simulink library "LopesDevelopmentLibrary"  (R2015b)
settings: Solver=ode45  StartTime=0.0  StopTime=10.0  RelTol=1e-3
values from neighbouring files (symbols this model uses):
  d2r = @(d) d*(pi/180)    [LopesDevelopmentLibrary_LoadParameters.m]
  ts = LopesParams.ts    [LopesDevelopmentLibrary_LoadParameters.m]
undefined symbols (not defined in the file or in its folder): anyParameterChanged, DiscIntNeverNeededParam, gcbh, LAP, LHF, LKF, LopesParams, macaddr, mxpcnetworkconfig, mxpcrtudprx, mxpcrtudptx, patientParametersChanged, port, PX, PZ, RAP, RHF, RKF, SelectorLOPESInSize, StrideTime_s, Time
undefined symbols (not defined in the file): LopesParamsSendDataArrayLen
libraries: LopesDevelopmentLibrary x327, simulink x100, dspmtrx3 x49, xpciplib x6, xpcnetworkbufferlib x5, dspsigops x4, dspstat3 x3, xpcethernetlib x2, visionstatistics x2, xpcseriallib x2, LopesDevelopmentLibraryTest x1, nmc x1
(part 6 of 12)

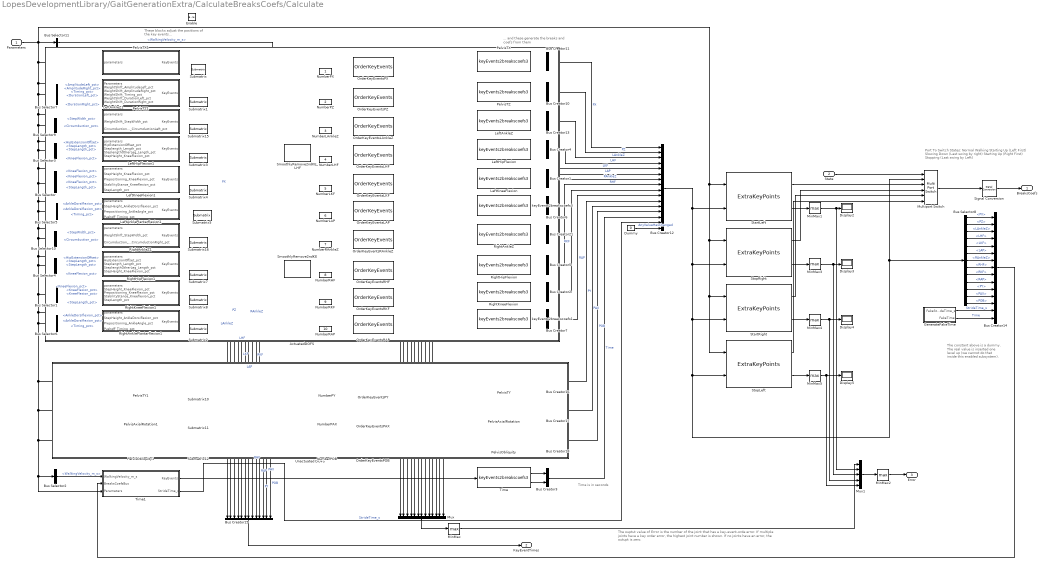
== system LopesDevelopmentLibrary/GaitGenerationExtra/CalculateBreaksCoefs/Calculate ==
  note: The ouptut value of Error is the number of the joint that has a key-event-orde  error.
      | If multiple joints have a key order error, the highest joint number is shown. If
      | no joints have an error, the outupt is zero.
  note: The constant above is
      | a dummy. The real value
      | is inserted one level up
      | (we cannot do that inside this
      | enabled subsystem).
  note: These blocks adjust the positions
      | of the key events...
  note: ... and these generate the breaks
      | and coefs from them
  note: Time is in seconds
  note: Port To Switch States:
      | Normal Walking
      | Starting Up (Left First)
      | Slowing Down (Last swing by right)
      | Starting Up (Right First)
      | Stopping (Last swing by Left)
  Parameters : Inport
  State : Inport  Port=2
  Enable : EnablePort
  ActuatedDOFS : Subsystem
      mask Display: disp('')
  Bus Creator{1..7,10..11,13,16..18,21} (14 alike) : BusCreator  Inputs=2
  Bus Creator12 : BusCreator  Inputs=16
  Bus Creator14 : BusCreator  Inputs=15
  Bus Creator15 : BusCreator  Inputs=13
  Bus Selector : BusSelector  OutputSignals=LeftStepHeight.KneeFlexion_pct,LeftPrepositioning.KneeFlexion_pct,LeftStabilityStance.KneeFlexion_pct,LeftSteplength.StepLength_pct
  Bus Selector1 : BusSelector  OutputSignals=RightStepHeight.KneeFlexion_pct,RightPrepositioning.KneeFlexion_pct,RightStabilityStance.KneeFlexion_pct,RightSteplength.StepLength_pct
  Bus Selector10 : BusSelector  OutputSignals=WeightShift.StepWidth_pct,RightCircumduction.Circumduction_pct
  Bus Selector11 : BusSelector  OutputSignals=General.WalkingVelocity_m_s
  Bus Selector2 : BusSelector  OutputSignals=General.WalkingVelocity_m_s
  Bus Selector3 : BusSelector  OutputSignals=General.HipExtensionOffset,LeftSteplength.StepLength_pct,RightSteplength.StepLength_pct,LeftStepHeight.KneeFlexion_pct
  Bus Selector4 : BusSelector  OutputSignals=General.HipExtensionOffset,RightSteplength.StepLength_pct,LeftSteplength.StepLength_pct,RightStepHeight.KneeFlexion_pct
  Bus Selector5 : BusSelector  OutputSignals=LeftStepHeight.AnkleDorsiflexion_pct,LeftPrepositioning.AnkleDorsiflexion_pct,LeftPushoff.Timing_pct
  Bus Selector6 : BusSelector  OutputSignals=RightStepHeight.AnkleDorsiflexion_pct,RightPrepositioning.AnkleDorsiflexion_pct,RightPushoff.Timing_pct
  Bus Selector7 : BusSelector  OutputSignals=WeightShift.AmplitudeLeft_pct,WeightShift.AmplitudeRight_pct,WeightShift.Timing_pct,WeightShift.DurationLeft_pct,WeightShift.DurationRight_pct
  Bus Selector8 : BusSelector  OutputSignals=PX,PZ,LAnkleZ,LHF,LKF,LAP,RAnkleZ,RHF,RKF,RAP,PY,PAX,POB
  Bus Selector9 : BusSelector  OutputSignals=WeightShift.StepWidth_pct,LeftCircumduction.Circumduction_pct
  Display{2..5} (4 alike) : Display
  Dummy : Constant  Value=0  OutDataTypeStr=double
  GenerateFakeTime : Subsystem
  LeftAnklePlantarflexion1 : Subsystem
  LeftAnkleZ : LopesDevelopmentLibrary/BlocksForInternalUse/GaitGeneration/keyEvents2breakscoefs3  SystemSampleTime=-1
  LeftAnkleZ1 : Subsystem
  LeftHipFlexion : LopesDevelopmentLibrary/BlocksForInternalUse/GaitGeneration/keyEvents2breakscoefs3  SystemSampleTime=-1
  LeftHipFlexion1 : Subsystem
  LeftKneeFlexion : LopesDevelopmentLibrary/BlocksForInternalUse/GaitGeneration/keyEvents2breakscoefs3  SystemSampleTime=-1
  LeftKneeFlexion1 : Subsystem
  MinMax{,1..5} (6 alike) : MinMax  Function=max
  Multiport Switch : MultiPortSwitch  Inputs=5
  Mux : Mux  Inputs=13
  Mux1 : Mux  Inputs=5
  NumberLAP : Constant  Value=6
  NumberLAnkleZ : Constant  Value=3
  NumberLHF : Constant  Value=4
  NumberLKF : Constant  Value=5
  NumberPAX : Constant  Value=12
  NumberPOB : Constant  Value=13
  NumberPX : Constant
  NumberPY : Constant  Value=11
  NumberPZ : Constant  Value=2
  NumberRAP : Constant  Value=10
  NumberRAnkleZ : Constant  Value=7
  NumberRHF : Constant  Value=8
  NumberRKF : Constant  Value=9
  OrderKeyEventsLAP : LopesDevelopmentLibrary/BlocksForInternalUse/GaitGeneration/OrderKeyEvents
  OrderKeyEventsLAnkleZ : LopesDevelopmentLibrary/BlocksForInternalUse/GaitGeneration/OrderKeyEvents
  OrderKeyEventsLHF : LopesDevelopmentLibrary/BlocksForInternalUse/GaitGeneration/OrderKeyEvents
  OrderKeyEventsLKF : LopesDevelopmentLibrary/BlocksForInternalUse/GaitGeneration/OrderKeyEvents
  OrderKeyEventsPAX : LopesDevelopmentLibrary/BlocksForInternalUse/GaitGeneration/OrderKeyEvents
  OrderKeyEventsPOB : LopesDevelopmentLibrary/BlocksForInternalUse/GaitGeneration/OrderKeyEvents
  OrderKeyEventsPX : LopesDevelopmentLibrary/BlocksForInternalUse/GaitGeneration/OrderKeyEvents
  OrderKeyEventsPY : LopesDevelopmentLibrary/BlocksForInternalUse/GaitGeneration/OrderKeyEvents
  OrderKeyEventsPZ : LopesDevelopmentLibrary/BlocksForInternalUse/GaitGeneration/OrderKeyEvents
  OrderKeyEventsRAP : LopesDevelopmentLibrary/BlocksForInternalUse/GaitGeneration/OrderKeyEvents
  OrderKeyEventsRAnkleZ : LopesDevelopmentLibrary/BlocksForInternalUse/GaitGeneration/OrderKeyEvents
  OrderKeyEventsRHF : LopesDevelopmentLibrary/BlocksForInternalUse/GaitGeneration/OrderKeyEvents
  OrderKeyEventsRKF : LopesDevelopmentLibrary/BlocksForInternalUse/GaitGeneration/OrderKeyEvents
  PelvisAxialRotation : LopesDevelopmentLibrary/BlocksForInternalUse/GaitGeneration/keyEvents2breakscoefs3  SystemSampleTime=-1
  PelvisAxialRotation1 : Subsystem
  PelvisObliquity : LopesDevelopmentLibrary/BlocksForInternalUse/GaitGeneration/keyEvents2breakscoefs3  SystemSampleTime=-1
  PelvisObliquity1 : Subsystem
  PelvisTX : LopesDevelopmentLibrary/BlocksForInternalUse/GaitGeneration/keyEvents2breakscoefs3  SystemSampleTime=-1
  PelvisTX1 : Subsystem
  PelvisTY : LopesDevelopmentLibrary/BlocksForInternalUse/GaitGeneration/keyEvents2breakscoefs3  SystemSampleTime=-1
  PelvisTY1 : Subsystem
  PelvisTZ : LopesDevelopmentLibrary/BlocksForInternalUse/GaitGeneration/keyEvents2breakscoefs3  SystemSampleTime=-1
  PelvisTZ1 : Subsystem
  RightAnklePlantarflexion1 : Subsystem
  RightAnkleZ : LopesDevelopmentLibrary/BlocksForInternalUse/GaitGeneration/keyEvents2breakscoefs3  SystemSampleTime=-1
  RightAnkleZ1 : Subsystem
  RightHipFlexion : LopesDevelopmentLibrary/BlocksForInternalUse/GaitGeneration/keyEvents2breakscoefs3  SystemSampleTime=-1
  RightHipFlexion1 : Subsystem
  RightKneeFlexion : LopesDevelopmentLibrary/BlocksForInternalUse/GaitGeneration/keyEvents2breakscoefs3  SystemSampleTime=-1
  RightKneeFlexion1 : Subsystem
  Signal Conversion : SignalConversion
  SmoothlyRemove2ndKE : LopesDevelopmentLibrary/BlocksForInternalUse/GaitGeneration/SmoothlyRemove2ndKE
  SmoothlyRemove2ndKE_LHF : LopesDevelopmentLibrary/BlocksForInternalUse/GaitGeneration/SmoothlyRemove2ndKE
  StartLeft : LopesDevelopmentLibrary/BlocksForInternalUse/GaitGenerationStartStop/ExtraKeyPoints   ExtraData='StartLeft'  ConnectionPoint=100  SetVelocity=0.3  SetStrideTime=2
  StartRight : LopesDevelopmentLibrary/BlocksForInternalUse/GaitGenerationStartStop/ExtraKeyPoints   ExtraData='StartRight'  ConnectionPoint=50  SetVelocity=0.3  SetStrideTime=2
  StopLeft : LopesDevelopmentLibrary/BlocksForInternalUse/GaitGenerationStartStop/ExtraKeyPoints   ExtraData='StopLeft'  ConnectionPoint=50  SetVelocity=0.3  SetStrideTime=2
  StopRight : LopesDevelopmentLibrary/BlocksForInternalUse/GaitGenerationStartStop/ExtraKeyPoints   ExtraData='StopRight'  ConnectionPoint=100  SetVelocity=0.3  SetStrideTime=2
  Submatrix{,1..5,7..8,10..12,15..16} (13 alike) : dspmtrx3/Submatrix  RowSpan=All rows  RowStartMode=First  RowStartIndex=1  RowEndMode=Last  RowEndIndex=1  ColSpan=One column  ColStartMode=First  ColStartIndex=1  ColEndMode=Last  ColEndIndex=1
  Time : LopesDevelopmentLibrary/BlocksForInternalUse/GaitGeneration/keyEvents2breakscoefs3  SystemSampleTime=-1
  Time1 : Subsystem
  Unactuated DOFS : Subsystem
      mask Display: disp('')
  keyEvents2breakscoefs1 : LopesDevelopmentLibrary/BlocksForInternalUse/GaitGeneration/keyEvents2breakscoefs3  SystemSampleTime=-1
  keyEvents2breakscoefs3 : LopesDevelopmentLibrary/BlocksForInternalUse/GaitGeneration/keyEvents2breakscoefs3  SystemSampleTime=-1
  BreaksCoefs : Outport  InitialOutput=0
  KeyEventTimes : Outport  Port=2
  Error : Outport  Port=3
  wires:
  Signal Conversion/1 -> BreaksCoefs/1
  OrderKeyEventsRKF/1 -> RightKneeFlexion/1
  OrderKeyEventsLHF/1 -> LeftHipFlexion/1
  Bus Selector7/5 -> PelvisTZ1/6(WeightShift_DurationRight_pct)  "<DurationRight_pct>"
  LeftHipFlexion1/1(KeyEvents) -> SmoothlyRemove2ndKE_LHF/1, Submatrix3/1
  LeftKneeFlexion/2 -> Bus Creator1/2
  LeftHipFlexion/1 -> Bus Creator4/1
  NumberRHF/1 -> OrderKeyEventsRHF/2
  LeftKneeFlexion/1 -> Bus Creator1/1
  MinMax/1 -> Mux1/1
  NumberRAnkleZ/1 -> OrderKeyEventsRAnkleZ/2
  OrderKeyEventsPOB/1 -> PelvisObliquity/1
  NumberLHF/1 -> OrderKeyEventsLHF/2
  OrderKeyEventsPY/1 -> PelvisTY/1
  NumberPZ/1 -> OrderKeyEventsPZ/2
  OrderKeyEventsPAX/1 -> PelvisAxialRotation/1
  LeftHipFlexion/2 -> Bus Creator4/2
  NumberLKF/1 -> OrderKeyEventsLKF/2
  Bus Selector3/4 -> LeftHipFlexion1/5(StepHeight_KneeFlexion_pct)  "<KneeFlexion_pct>"
  NumberRKF/1 -> OrderKeyEventsRKF/2
  Bus Selector3/3 -> LeftHipFlexion1/4(SteplengthOtherLeg_Length_pct)  "<StepLength_pct>"
  Bus Selector3/2 -> LeftHipFlexion1/3(Steplength_Length_pct)  "<StepLength_pct>"
  Dummy/1 -> Bus Creator12/16  "AnyValueHasChanged"
  RightHipFlexion1/1(KeyEvents) -> Submatrix7/1, SmoothlyRemove2ndKE/1
  RightKneeFlexion1/1(KeyEvents) -> OrderKeyEventsRKF/1, Submatrix8/1
  PelvisTX/2 -> Bus Creator11/2
  Bus Creator2/1 -> Bus Creator12/9  "RKF"
  PelvisTX/1 -> Bus Creator11/1
  Bus Creator1/1 -> Bus Creator12/5  "LKF"
  RightHipFlexion/2 -> Bus Creator5/2
  GenerateFakeTime/1(FakeStrideTime_s) -> Bus Creator14/14  "StrideTime_s"
  Bus Selector7/3 -> PelvisTZ1/4(WeightShift_Timing_pct)  "<Timing_pct>"
  LeftKneeFlexion1/1(KeyEvents) -> OrderKeyEventsLKF/1, Submatrix4/1
  Bus Selector7/1 -> PelvisTZ1/2(WeightShift_AmplitudeLeft_pct)  "<AmplitudeLeft_pct>"
  Bus Creator5/1 -> Bus Creator12/8  "RHF"
  Bus Selector7/4 -> PelvisTZ1/5(WeightShift_DurationLeft_pct)  "<DurationLeft_pct>"
  Bus Selector/1 -> LeftKneeFlexion1/2(StepHeight_KneeFlexion_pct)  "<KneeFlexion_pct>"
  Bus Selector4/4 -> RightHipFlexion1/5(StepHeight_KneeFlexion_pct)  "<KneeFlexion_pct>"
  PelvisTX1/1(KeyEvents) -> Submatrix/1, OrderKeyEventsPX/1
  Bus Creator15/1 -> KeyEventTimes/1
  Bus Creator10/1 -> Bus Creator12/2  "PZ"
  Bus Creator11/1 -> Bus Creator12/1  "PX"
  Bus Creator4/1 -> Bus Creator12/4  "LHF"
  Bus Selector4/3 -> RightHipFlexion1/4(SteplengthOtherLeg_Length_pct)  "<StepLength_pct>"
  Bus Selector4/2 -> RightHipFlexion1/3(Steplength_Length_pct)  "<StepLength_pct>"
  PelvisTZ1/1(KeyEvents) -> OrderKeyEventsPZ/1, Submatrix1/1
  PelvisTZ/1 -> Bus Creator10/1
  PelvisTZ/2 -> Bus Creator10/2
  Bus Selector1/4 -> RightKneeFlexion1/5(StepLength_pct)  "<StepLength_pct>"
  SmoothlyRemove2ndKE/1 -> OrderKeyEventsRHF/1
  Bus Selector4/1 -> RightHipFlexion1/2(HipExtensionOffset_pct)  "<HipExtensionOffset>"
  Submatrix10/1 -> Bus Creator15/11  "PY"
  Time1/2(StrideTime_s) -> Bus Creator12/15  "StrideTime_s"
  SmoothlyRemove2ndKE_LHF/1 -> OrderKeyEventsLHF/1
  Bus Selector3/1 -> LeftHipFlexion1/2(HipExtensionOffset_pct)  "<HipExtensionOffset>"
  Bus Selector1/3 -> RightKneeFlexion1/4(StabilityStance_Kneeflexion_pct)  "<KneeFlexion_pct>"
  Bus Selector1/1 -> RightKneeFlexion1/2(StepHeight_KneeFlexion_pct)  "<KneeFlexion_pct>"
  Bus Selector9/2 -> LeftAnkleZ1/3(Circumduction_CircumductionLeft_pct)  "<Circumduction_pct>"
  Bus Selector9/1 -> LeftAnkleZ1/2(WeightShift_StepWidth_pct)  "<StepWidth_pct>"
  NumberLAnkleZ/1 -> OrderKeyEventsLAnkleZ/2
  Bus Selector8/1 -> Bus Creator14/1  "<PX>"
  Bus Selector10/1 -> RightAnkleZ1/2(WeightShift_StepWidth_pct)  "<StepWidth_pct>"
  NumberPX/1 -> OrderKeyEventsPX/2
  Bus Selector10/2 -> RightAnkleZ1/3(Circumduction_CircumductionRight_pct)  "<Circumduction_pct>"
  Bus Selector/4 -> LeftKneeFlexion1/5(StepLength_pct)  "<StepLength_pct>"
  OrderKeyEventsRAnkleZ/1 -> RightAnkleZ/1
  Bus Creator21/1 -> Bus Creator12/7  "RAnkleZ"
  Bus Selector1/2 -> RightKneeFlexion1/3(Prepositioning_KneeFlexion_pct)  "<KneeFlexion_pct>"
  Mux/1 -> MinMax/1
  Bus Selector7/2 -> PelvisTZ1/3(WeightShift_AmplitudeRight_pct)  "<AmplitudeRight_pct>"
  Bus Selector/2 -> LeftKneeFlexion1/3(Prepositioning_KneeFlexion_pct)  "<KneeFlexion_pct>"
  Bus Creator13/1 -> Bus Creator12/3  "LAnkleZ"
  Bus Selector8/2 -> Bus Creator14/2  "<PZ>"
  Bus Selector/3 -> LeftKneeFlexion1/4(StabilityStance_Kneeflexion_pct)  "<KneeFlexion_pct>"
  Bus Selector8/8 -> Bus Creator14/8  "<RHF>"
  LeftAnkleZ/2 -> Bus Creator13/2
  LeftAnkleZ1/1(KeyEvents) -> Submatrix15/1, OrderKeyEventsLAnkleZ/1
  LeftAnkleZ/1 -> Bus Creator13/1
  RightAnkleZ/2 -> Bus Creator21/2
  RightAnkleZ/1 -> Bus Creator21/1
  RightAnkleZ1/1(KeyEvents) -> Submatrix16/1, OrderKeyEventsRAnkleZ/1
  Bus Selector8/12 -> Bus Creator14/12  "<PAX>"
  OrderKeyEventsLAnkleZ/1 -> LeftAnkleZ/1
  Submatrix11/1 -> Bus Creator15/12  "PAX"
  Time/1 -> Bus Creator3/1
  PelvisTY/1 -> Bus Creator16/1
  Bus Selector8/4 -> Bus Creator14/4  "<LHF>"
  Bus Selector8/7 -> Bus Creator14/7  "<RAnkleZ>"
  Bus Selector8/11 -> Bus Creator14/11  "<PY>"
  OrderKeyEventsLAnkleZ/2 -> Mux/3
  Bus Selector8/13 -> Bus Creator14/13  "<POB>"
  Submatrix12/1 -> Bus Creator15/13  "POB"
  Bus Selector8/9 -> Bus Creator14/9  "<RKF>"
  Submatrix8/1 -> Bus Creator15/9  "RKF"
  Submatrix7/1 -> Bus Creator15/8  "RHF"
  Bus Selector8/5 -> Bus Creator14/5  "<LKF>"
  PelvisObliquity1/1(KeyEvents) -> Submatrix12/1, OrderKeyEventsPOB/1
  Bus Selector11/1 -> SmoothlyRemove2ndKE/2, SmoothlyRemove2ndKE_LHF/2  "<WalkingVelocity_m_s>"
  PelvisTY1/1(KeyEvents) -> OrderKeyEventsPY/1, Submatrix10/1
  OrderKeyEventsPZ/2 -> Mux/2
  Submatrix16/1 -> Bus Creator15/7  "RAnkleZ"
  GenerateFakeTime/2(FakeTime) -> Bus Creator14/15  "Time"
  OrderKeyEventsRHF/2 -> Mux/8
  NumberPOB/1 -> OrderKeyEventsPOB/2
  OrderKeyEventsLKF/2 -> Mux/5
  NumberPY/1 -> OrderKeyEventsPY/2
  OrderKeyEventsRAnkleZ/2 -> Mux/7
  Bus Creator16/1 -> Bus Creator12/11  "PY"
  Submatrix/1 -> Bus Creator15/1  "PX"
  Submatrix15/1 -> Bus Creator15/3  "LAnkleZ"
  Submatrix3/1 -> Bus Creator15/4  "LHF"
  Submatrix1/1 -> Bus Creator15/2  "PZ"
  OrderKeyEventsLHF/2 -> Mux/4
  Submatrix4/1 -> Bus Creator15/5  "LKF"
  OrderKeyEventsRKF/2 -> Mux/9
  OrderKeyEventsPY/2 -> Mux/11
  OrderKeyEventsPOB/2 -> Mux/13
  OrderKeyEventsPX/2 -> Mux/1
  OrderKeyEventsPAX/2 -> Mux/12
  Bus Selector8/3 -> Bus Creator14/3  "<LAnkleZ>"
  PelvisTY/2 -> Bus Creator16/2
  OrderKeyEventsRHF/1 -> RightHipFlexion/1
  Time/2 -> Bus Creator3/2
  Bus Creator14/1 -> Time1/2(BreaksCoefsBus)
  RightHipFlexion/1 -> Bus Creator5/1
  OrderKeyEventsPX/1 -> PelvisTX/1
  OrderKeyEventsLKF/1 -> LeftKneeFlexion/1
  OrderKeyEventsPZ/1 -> PelvisTZ/1
  RightKneeFlexion/1 -> Bus Creator2/1
  Time1/1(KeyEvents) -> Time/1
  Bus Selector2/1 -> Time1/1(WalkingVelocity_m_s)  "<WalkingVelocity_m_s>"
  RightKneeFlexion/2 -> Bus Creator2/2
  PelvisObliquity/2 -> Bus Creator18/2
  Bus Creator17/1 -> Bus Creator12/12  "PAX"
  PelvisAxialRotation1/1(KeyEvents) -> Submatrix11/1, OrderKeyEventsPAX/1
  PelvisAxialRotation/2 -> Bus Creator17/2
  PelvisAxialRotation/1 -> Bus Creator17/1
  NumberPAX/1 -> OrderKeyEventsPAX/2
  Bus Creator18/1 -> Bus Creator12/13  "POB"
  PelvisObliquity/1 -> Bus Creator18/1
  Bus Creator3/1 -> Bus Creator12/14  "Time"
  OrderKeyEventsLAP/1 -> keyEvents2breakscoefs3/1
  OrderKeyEventsRAP/1 -> keyEvents2breakscoefs1/1
  keyEvents2breakscoefs3/1 -> Bus Creator6/1
  keyEvents2breakscoefs3/2 -> Bus Creator6/2
  Bus Creator6/1 -> Bus Creator12/6  "LAP"
  keyEvents2breakscoefs1/2 -> Bus Creator7/2
  keyEvents2breakscoefs1/1 -> Bus Creator7/1
  Bus Creator7/1 -> Bus Creator12/10  "RAP"
  Bus Selector8/10 -> Bus Creator14/10  "<RAP>"
  Bus Selector8/6 -> Bus Creator14/6  "<LAP>"
  OrderKeyEventsRAP/2 -> Mux/10
  OrderKeyEventsLAP/2 -> Mux/6
  NumberLAP/1 -> OrderKeyEventsLAP/2
  NumberRAP/1 -> OrderKeyEventsRAP/2
  RightAnklePlantarflexion1/1(KeyEvents) -> Submatrix2/1, OrderKeyEventsRAP/1
  Submatrix2/1 -> Bus Creator15/10  "RAP"
  LeftAnklePlantarflexion1/1(KeyEvents) -> OrderKeyEventsLAP/1, Submatrix5/1
  Submatrix5/1 -> Bus Creator15/6  "LAP"
  Bus Selector5/1 -> LeftAnklePlantarflexion1/2(StepHeight_AnkleDorsiflexion_pct)  "<AnkleDorsiflexion_pct>"
  Bus Selector5/2 -> LeftAnklePlantarflexion1/3(Prepositioning_AnkleAngle_pct)  "<AnkleDorsiflexion_pct>"
  Bus Selector5/3 -> LeftAnklePlantarflexion1/4(Pushoff_Timing_pct)  "<Timing_pct>"
  Bus Selector6/3 -> RightAnklePlantarflexion1/4(Pushoff_Timing_pct)  "<Timing_pct>"
  Bus Selector6/2 -> RightAnklePlantarflexion1/3(Prepositioning_AnkleAngle_pct)  "<AnkleDorsiflexion_pct>"
  Bus Selector6/1 -> RightAnklePlantarflexion1/2(StepHeight_AnkleDorsiflexion_pct)  "<AnkleDorsiflexion_pct>"
  MinMax5/1 -> Mux1/5, Display5/1
  MinMax4/1 -> Mux1/4, Display4/1
  StopLeft/2 -> MinMax5/1
  StartRight/2 -> MinMax4/1
  StopLeft/1 -> Multiport Switch/6
  StartRight/1 -> Multiport Switch/5
  StopRight/1 -> Multiport Switch/4
  MinMax3/1 -> Mux1/3, Display3/1
  StopRight/2 -> MinMax3/1
  StartLeft/1 -> Multiport Switch/3
  State/1 -> Multiport Switch/1
  MinMax1/1 -> Mux1/2, Display2/1
  StartLeft/2 -> MinMax1/1
  Parameters/1 -> Bus Selector11/1, StartLeft/1, StopRight/1, StartRight/1, StopLeft/1, Bus Selector5/1, RightAnklePlantarflexion1/1(parameters), Bus Selector6/1, Time1/3(Parameters), Bus Selector2/1, PelvisObliquity1/1(parameters), PelvisAxialRotation1/1(parameters), PelvisTY1/1(parameters), Bus Selector1/1, Bus Selector4/1, RightHipFlexion1/1(parameters), RightKneeFlexion1/1(parameters), Bus Selector10/1, RightAnkleZ1/1(parameters), LeftAnklePlantarflexion1/1(parameters), Bus Selector/1, LeftKneeFlexion1/1(parameters), Bus Selector3/1, LeftHipFlexion1/1(parameters), Bus Selector9/1, LeftAnkleZ1/1(parameters), Bus Selector7/1, PelvisTZ1/1(Parameters), PelvisTX1/1(parameters)
  Multiport Switch/1 -> Signal Conversion/1
  Mux1/1 -> MinMax2/1
  MinMax2/1 -> Error/1
  Bus Creator12/1 -> StartLeft/2, Bus Selector8/1, Multiport Switch/2, StopLeft/2, StartRight/2, StopRight/2

== system LopesDevelopmentLibrary/GaitGenerationExtra/GaitGenerationAndAnalysis/DesiredStateToSetState ==
  DesiredState : Inport
  Add : Sum  Inputs=5
  Add2 : Sum
  Compare To Constant1 : simulink/Logic and Bit Operations/Compare To Constant  relop=<  const=200  OutDataTypeStr=boolean
  Compare To Constant10 : simulink/Logic and Bit Operations/Compare To Constant  relop===  const=302  OutDataTypeStr=boolean
  Compare To Constant2 : simulink/Logic and Bit Operations/Compare To Constant  relop===  const=501  OutDataTypeStr=boolean
  Compare To Constant3 : simulink/Logic and Bit Operations/Compare To Constant  relop===  const=201  OutDataTypeStr=boolean
  Compare To Constant4 : simulink/Logic and Bit Operations/Compare To Constant  relop===  const=502  OutDataTypeStr=boolean
  Compare To Constant5 : simulink/Logic and Bit Operations/Compare To Constant  relop=>=  const=100  OutDataTypeStr=boolean
  Compare To Constant6 : simulink/Logic and Bit Operations/Compare To Constant  relop===  const=202  OutDataTypeStr=boolean
  Compare To Constant7 : simulink/Logic and Bit Operations/Compare To Constant  relop===  const=402  OutDataTypeStr=boolean
  Compare To Constant8 : simulink/Logic and Bit Operations/Compare To Constant  relop===  const=401  OutDataTypeStr=boolean
  Compare To Constant9 : simulink/Logic and Bit Operations/Compare To Constant  relop===  const=301  OutDataTypeStr=boolean
  Gain : Gain
  Gain1 : Gain  Gain=2
  Gain2 : Gain  Gain=4
  Gain3 : Gain  Gain=3
  Gain4 : Gain  Gain=5
  Gain7 : Gain  Gain=50  OutDataTypeStr=double
  Gain8 : Gain  Gain=0  OutDataTypeStr=double
  Logical Operator : Logic  AllPortsSameDT=off  OutDataTypeStr=boolean
  Logical Operator{1..10} (10 alike) : Logic  Operator=OR  AllPortsSameDT=off  OutDataTypeStr=boolean
  Unit Delay : UnitDelay  SampleTime=-1
  Unit Delay1 : UnitDelay  SampleTime=-1
  Unit Delay2 : UnitDelay  SampleTime=-1
  Unit Delay3 : UnitDelay  InitialCondition=2  SampleTime=-1
  Unit Delay4 : UnitDelay  InitialCondition=2  SampleTime=-1
  SetState : Outport
  Reset : Outport  Port=2
  ResetPercentage : Outport  Port=3
  FinalState : Outport  Port=4
  wires:
  Compare To Constant1/1 -> Logical Operator/2
  Compare To Constant5/1 -> Logical Operator/1
  Compare To Constant2/1 -> Logical Operator8/1, Logical Operator1/2
  Compare To Constant3/1 -> Logical Operator1/1
  Compare To Constant4/1 -> Logical Operator9/1, Logical Operator2/2
  Compare To Constant6/1 -> Logical Operator2/1
  Compare To Constant8/1 -> Logical Operator8/2, Logical Operator3/1
  Compare To Constant9/1 -> Logical Operator7/1, Logical Operator5/1, Logical Operator3/2
  Compare To Constant7/1 -> Logical Operator9/2, Logical Operator4/1
  DesiredState/1 -> Compare To Constant2/1, Compare To Constant1/1, Compare To Constant5/1, Compare To Constant3/1, Compare To Constant6/1, Compare To Constant7/1, Compare To Constant10/1, Compare To Constant9/1, Compare To Constant8/1, Compare To Constant4/1
  Compare To Constant10/1 -> Logical Operator7/2, Logical Operator6/2, Logical Operator4/2
  Logical Operator1/1 -> Gain1/1
  Logical Operator/1 -> Gain/1
  Logical Operator2/1 -> Gain2/1
  Logical Operator3/1 -> Gain3/1
  Logical Operator4/1 -> Gain4/1
  Gain/1 -> Add/1
  Gain1/1 -> Add/2
  Gain2/1 -> Add/3
  Gain3/1 -> Add/4
  Gain4/1 -> Add/5
  Add/1 -> Unit Delay4/1
  Logical Operator9/1 -> Logical Operator6/1, Logical Operator10/2
  Logical Operator8/1 -> Logical Operator10/1, Logical Operator5/2
  Unit Delay4/1 -> Unit Delay3/1
  Unit Delay3/1 -> SetState/1
  Gain8/1 -> Add2/2
  Gain7/1 -> Add2/1
  Logical Operator10/1 -> Unit Delay2/1
  Add2/1 -> Unit Delay/1
  Logical Operator5/1 -> Gain7/1
  Logical Operator6/1 -> Gain8/1
  Unit Delay/1 -> Unit Delay1/1
  Unit Delay1/1 -> ResetPercentage/1
  Unit Delay2/1 -> Reset/1
  Logical Operator7/1 -> FinalState/1

== system LopesDevelopmentLibrary/GaitGenerationExtra/GaitParameters/AssignChangedElements ==
  note: This block checks whether any of the parameters changed during
      | this sampletime, and assigns the correct values to the anyParameterChanged
      | and patientParametersChanged bus elements.
  BusIn : Inport
  PatientParametersChanged : Inport  Port=2
  AnyChanged : LopesDevelopmentLibrary/Various/AnyChanged
  Bus Assignment : BusAssignment  AssignedSignals=patientParametersChanged,anyParameterChanged
  Bus Selector : BusSelector  OutputSignals=Patient,General,WeightShift,LeftStepHeight,RightStepHeight,LeftCircumduction,RightCircumduction,LeftStabilityStance,RightStabilityStance,LeftPrepositioning,RightPrepositioning,LeftSteplength,RightSteplength  OutputAsBus=on
  Data Type Conversion2 : DataTypeConversion
  Logical Operator : Logic  Operator=OR  AllPortsSameDT=off  OutDataTypeStr=boolean
  BusOut : Outport
  Changed : Outport  Port=2
  wires:
  Data Type Conversion2/1 -> Changed/1
  Bus Assignment/1 -> BusOut/1
  Bus Selector/1 -> AnyChanged/1
  PatientParametersChanged/1 -> Logical Operator/1, Bus Assignment/2
  BusIn/1 -> Bus Selector/1, Bus Assignment/1
  Logical Operator/1 -> Bus Assignment/3, Data Type Conversion2/1
  AnyChanged/1 -> Logical Operator/2

== system LopesDevelopmentLibrary/GaitGenerationExtra/GaitParameters/Circumduction ==

== system LopesDevelopmentLibrary/GaitGenerationExtra/GaitParameters/General ==

== system LopesDevelopmentLibrary/GaitGenerationExtra/GaitParameters/Prepositioning ==

== system LopesDevelopmentLibrary/GaitGenerationExtra/GaitParameters/Pushoff ==

== system LopesDevelopmentLibrary/GaitGenerationExtra/GaitParameters/RateLimitCircumduction ==
  GeneralGF : Inport
  In2 : Inport  Port=2
  In3 : Inport  Port=3
  In4 : Inport  Port=4
  In5 : Inport  Port=5
  In6 : Inport  Port=6
  In7 : Inport  Port=7
  Bus Creator1 : BusCreator  Inputs=2
  Bus Creator2 : BusCreator  Inputs=2
  Rate Limiter : RateLimiter  RisingSlewLimit=100  FallingSlewLimit=-100  SampleTimeMode=inherited
  Rate Limiter1 : RateLimiter  RisingSlewLimit=50  FallingSlewLimit=-50  SampleTimeMode=inherited
  Rate Limiter2 : RateLimiter  RisingSlewLimit=50  FallingSlewLimit=-50  SampleTimeMode=inherited
  Rate Limiter7 : RateLimiter  RisingSlewLimit=100  FallingSlewLimit=-100  SampleTimeMode=inherited
  Switch : Switch  Criteria=u2 ~= 0
  Switch1 : Switch  Criteria=u2 ~= 0
  Left : Outport
  Right : Outport  Port=2
  wires:
  Bus Creator1/1 -> Left/1
  Rate Limiter1/1 -> Bus Creator1/2  "Circumduction_pct"
  Rate Limiter/1 -> Bus Creator1/1  "GuidanceForce_pct"
  Switch1/1 -> Rate Limiter7/1
  In2/1 -> Switch/2
  In6/1 -> Switch1/1
  In3/1 -> Switch/1
  In5/1 -> Switch1/2
  In7/1 -> Rate Limiter2/1
  Switch/1 -> Rate Limiter/1  "GuidanceForce_pct"
  In4/1 -> Rate Limiter1/1
  GeneralGF/1 -> Switch/3, Switch1/3
  Rate Limiter2/1 -> Bus Creator2/2  "Circumduction_pct"
  Rate Limiter7/1 -> Bus Creator2/1  "GuidanceForce_pct"
  Bus Creator2/1 -> Right/1

== system LopesDevelopmentLibrary/GaitGenerationExtra/GaitParameters/RateLimitGeneral ==
  In1 : Inport
  In2 : Inport  Port=2
  In3 : Inport  Port=3
  Bus Creator1 : BusCreator  Inputs=3
  ConvertToKm_h : Gain  Gain=3.6
  Rate Limiter1 : RateLimiter  RisingSlewLimit=50  FallingSlewLimit=-50  SampleTimeMode=inherited
  Rate Limiter2 : RateLimiter  RisingSlewLimit=0.1  FallingSlewLimit=-0.1  SampleTimeMode=inherited
  Rate Limiter3 : RateLimiter  RisingSlewLimit=20  FallingSlewLimit=-20  SampleTimeMode=inherited
  km_h : Outport
  General : Outport  Port=2
  wires:
  Bus Creator1/1 -> General/1  "General"
  In3/1 -> Rate Limiter1/1
  In2/1 -> Rate Limiter3/1
  In1/1 -> ConvertToKm_h/1, Rate Limiter2/1
  ConvertToKm_h/1 -> km_h/1
  Rate Limiter2/1 -> Bus Creator1/1  "WalkingVelocity_m_s"
  Rate Limiter3/1 -> Bus Creator1/2  "GuidanceForce_pct"
  Rate Limiter1/1 -> Bus Creator1/3  "HipExtensionOffset"

== system LopesDevelopmentLibrary/GaitGenerationExtra/GaitParameters/RateLimitPrepositioning ==
  GeneralGF : Inport
  In2 : Inport  Port=2
  In3 : Inport  Port=3
  In4 : Inport  Port=4
  In1 : Inport  Port=5
  In5 : Inport  Port=6
  In6 : Inport  Port=7
  In7 : Inport  Port=8
  In8 : Inport  Port=9
  Bus Creator1 : BusCreator  Inputs=3
  Bus Creator2 : BusCreator  Inputs=3
  Rate Limiter : RateLimiter  RisingSlewLimit=100  FallingSlewLimit=-100  SampleTimeMode=inherited
  Rate Limiter{1..4} (4 alike) : RateLimiter  RisingSlewLimit=50  FallingSlewLimit=-50  SampleTimeMode=inherited
  Rate Limiter7 : RateLimiter  RisingSlewLimit=100  FallingSlewLimit=-100  SampleTimeMode=inherited
  Switch : Switch  Criteria=u2 ~= 0
  Switch1 : Switch  Criteria=u2 ~= 0
  Left : Outport
  Right : Outport  Port=2
  wires:
  Bus Creator1/1 -> Left/1
  Rate Limiter1/1 -> Bus Creator1/2  "KneeFlexion_pct"
  Rate Limiter/1 -> Bus Creator1/1  "GuidanceForce_pct"
  Switch1/1 -> Rate Limiter7/1
  In2/1 -> Switch/2
  In6/1 -> Switch1/1
  In3/1 -> Switch/1
  In5/1 -> Switch1/2
  In7/1 -> Rate Limiter2/1
  Switch/1 -> Rate Limiter/1  "GuidanceForce_pct"
  In4/1 -> Rate Limiter1/1
  GeneralGF/1 -> Switch/3, Switch1/3
  Rate Limiter2/1 -> Bus Creator2/2  "KneeFlexion_pct"
  Rate Limiter7/1 -> Bus Creator2/1  "GuidanceForce_pct"
  Bus Creator2/1 -> Right/1
  Rate Limiter3/1 -> Bus Creator1/3  "AnkleDorsiflexion_pct"
  In1/1 -> Rate Limiter3/1
  Rate Limiter4/1 -> Bus Creator2/3  "AnkleDorsiflexion_pct"
  In8/1 -> Rate Limiter4/1

== system LopesDevelopmentLibrary/GaitGenerationExtra/GaitParameters/RateLimitPushoff ==
  GeneralGF : Inport
  In2 : Inport  Port=2
  In3 : Inport  Port=3
  In4 : Inport  Port=4
  In1 : Inport  Port=5
  In5 : Inport  Port=6
  In6 : Inport  Port=7
  In7 : Inport  Port=8
  In8 : Inport  Port=9
  Bus Creator1 : BusCreator  Inputs=3
  Bus Creator2 : BusCreator  Inputs=3
  Rate Limiter : RateLimiter  RisingSlewLimit=100  FallingSlewLimit=-100  SampleTimeMode=inherited
  Rate Limiter1 : RateLimiter  RisingSlewLimit=50  FallingSlewLimit=-50  SampleTimeMode=inherited
  Rate Limiter2 : RateLimiter  RisingSlewLimit=50  FallingSlewLimit=-50  SampleTimeMode=inherited
  Rate Limiter3 : RateLimiter  RisingSlewLimit=10  FallingSlewLimit=-10  SampleTimeMode=inherited
  Rate Limiter4 : RateLimiter  RisingSlewLimit=10  FallingSlewLimit=-10  SampleTimeMode=inherited
  Rate Limiter7 : RateLimiter  RisingSlewLimit=100  FallingSlewLimit=-100  SampleTimeMode=inherited
  Switch : Switch  Criteria=u2 ~= 0
  Switch1 : Switch  Criteria=u2 ~= 0
  Left : Outport
  Right : Outport  Port=2
  wires:
  In8/1 -> Rate Limiter4/1
  Rate Limiter4/1 -> Bus Creator2/3  "Timing_pct"
  In1/1 -> Rate Limiter3/1
  Rate Limiter3/1 -> Bus Creator1/3  "Timing_pct"
  Bus Creator2/1 -> Right/1
  Rate Limiter7/1 -> Bus Creator2/1  "GuidanceForce_pct"
  Rate Limiter2/1 -> Bus Creator2/2  "HipExtension_pct"
  GeneralGF/1 -> Switch1/3, Switch/3
  In4/1 -> Rate Limiter1/1
  Switch/1 -> Rate Limiter/1  "GuidanceForce_pct"
  In7/1 -> Rate Limiter2/1
  In5/1 -> Switch1/2
  In3/1 -> Switch/1
  In6/1 -> Switch1/1
  In2/1 -> Switch/2
  Switch1/1 -> Rate Limiter7/1
  Rate Limiter/1 -> Bus Creator1/1  "GuidanceForce_pct"
  Rate Limiter1/1 -> Bus Creator1/2  "HipExtension_pct"
  Bus Creator1/1 -> Left/1

== system LopesDevelopmentLibrary/GaitGenerationExtra/GaitParameters/RateLimitStabilityStance ==
  GeneralGF : Inport
  In2 : Inport  Port=2
  In3 : Inport  Port=3
  In4 : Inport  Port=4
  In5 : Inport  Port=5
  In6 : Inport  Port=6
  In7 : Inport  Port=7
  Bus Creator1 : BusCreator  Inputs=2
  Bus Creator2 : BusCreator  Inputs=2
  Rate Limiter : RateLimiter  RisingSlewLimit=100  FallingSlewLimit=-100  SampleTimeMode=inherited
  Rate Limiter1 : RateLimiter  RisingSlewLimit=50  FallingSlewLimit=-50  SampleTimeMode=inherited
  Rate Limiter2 : RateLimiter  RisingSlewLimit=50  FallingSlewLimit=-50  SampleTimeMode=inherited
  Rate Limiter7 : RateLimiter  RisingSlewLimit=100  FallingSlewLimit=-100  SampleTimeMode=inherited
  Switch : Switch  Criteria=u2 ~= 0
  Switch1 : Switch  Criteria=u2 ~= 0
  Left : Outport
  Right : Outport  Port=2
  wires:
  Bus Creator2/1 -> Right/1
  Rate Limiter7/1 -> Bus Creator2/1  "GuidanceForce_pct"
  Rate Limiter2/1 -> Bus Creator2/2  "KneeFlexion_pct"
  GeneralGF/1 -> Switch1/3, Switch/3
  In4/1 -> Rate Limiter1/1
  Switch/1 -> Rate Limiter/1  "GuidanceForce_pct"
  In7/1 -> Rate Limiter2/1
  In5/1 -> Switch1/2
  In3/1 -> Switch/1
  In6/1 -> Switch1/1
  In2/1 -> Switch/2
  Switch1/1 -> Rate Limiter7/1
  Rate Limiter/1 -> Bus Creator1/1  "GuidanceForce_pct"
  Rate Limiter1/1 -> Bus Creator1/2  "KneeFlexion_pct"
  Bus Creator1/1 -> Left/1

== system LopesDevelopmentLibrary/GaitGenerationExtra/GaitParameters/RateLimitStepHeight ==
  GeneralGF : Inport
  In2 : Inport  Port=2
  In3 : Inport  Port=3
  In1 : Inport  Port=4
  In4 : Inport  Port=5
  In5 : Inport  Port=6
  In6 : Inport  Port=7
  In8 : Inport  Port=8
  In7 : Inport  Port=9
  Bus Creator1 : BusCreator  Inputs=3
  Bus Creator2 : BusCreator  Inputs=3
  Rate Limiter : RateLimiter  RisingSlewLimit=100  FallingSlewLimit=-100  SampleTimeMode=inherited
  Rate Limiter1 : RateLimiter  RisingSlewLimit=50  FallingSlewLimit=-50  SampleTimeMode=inherited
  Rate Limiter2 : RateLimiter  RisingSlewLimit=50  FallingSlewLimit=-50  SampleTimeMode=inherited
  Rate Limiter3 : RateLimiter  RisingSlewLimit=100  FallingSlewLimit=-100  SampleTimeMode=inherited
  Rate Limiter4 : RateLimiter  RisingSlewLimit=50  FallingSlewLimit=-50  SampleTimeMode=inherited
  Rate Limiter7 : RateLimiter  RisingSlewLimit=100  FallingSlewLimit=-100  SampleTimeMode=inherited
  Switch : Switch  Criteria=u2 ~= 0
  Switch1 : Switch  Criteria=u2 ~= 0
  Left : Outport
  Right : Outport  Port=2
  wires:
  Bus Creator2/1 -> Right/1
  Rate Limiter7/1 -> Bus Creator2/1  "GuidanceForce_pct"
  Rate Limiter2/1 -> Bus Creator2/3  "KneeFlexion_pct"
  GeneralGF/1 -> Switch/3, Switch1/3
  In4/1 -> Rate Limiter1/1
  Switch/1 -> Rate Limiter/1  "GuidanceForce_pct"
  In7/1 -> Rate Limiter2/1
  In5/1 -> Switch1/2
  In3/1 -> Switch/1
  In6/1 -> Switch1/1
  In2/1 -> Switch/2
  Switch1/1 -> Rate Limiter7/1
  Rate Limiter/1 -> Bus Creator1/1  "GuidanceForce_pct"
  Rate Limiter1/1 -> Bus Creator1/3  "KneeFlexion_pct"
  Bus Creator1/1 -> Left/1
  Rate Limiter3/1 -> Bus Creator1/2  "AnkleDorsiflexion_pct"
  In1/1 -> Rate Limiter3/1
  Rate Limiter4/1 -> Bus Creator2/2  "AnkleDorsiflexion_pct"
  In8/1 -> Rate Limiter4/1

== system LopesDevelopmentLibrary/GaitGenerationExtra/GaitParameters/RateLimitStepLength ==
  GeneralGF : Inport
  In2 : Inport  Port=2
  In3 : Inport  Port=3
  In4 : Inport  Port=4
  Bus Creator1 : BusCreator  Inputs=2
  Rate Limiter : RateLimiter  RisingSlewLimit=100  FallingSlewLimit=-100  SampleTimeMode=inherited
  Rate Limiter1 : RateLimiter  RisingSlewLimit=5  FallingSlewLimit=-5  SampleTimeMode=inherited
  Switch : Switch  Criteria=u2 ~= 0
  StepLength : Outport
  wires:
  GeneralGF/1 -> Switch/3
  In4/1 -> Rate Limiter1/1
  Switch/1 -> Rate Limiter/1  "GuidanceForce_pct"
  In3/1 -> Switch/1
  In2/1 -> Switch/2
  Rate Limiter/1 -> Bus Creator1/1  "GuidanceForce_pct"
  Rate Limiter1/1 -> Bus Creator1/2  "StepLength_pct"
  Bus Creator1/1 -> StepLength/1

== system LopesDevelopmentLibrary/GaitGenerationExtra/GaitParameters/RateLimitWeightShift ==
  GeneralGF : Inport
  In2 : Inport  Port=2
  In3 : Inport  Port=3
  In4 : Inport  Port=4
  In5 : Inport  Port=5
  In6 : Inport  Port=6
  In7 : Inport  Port=7
  In8 : Inport  Port=8
  In9 : Inport  Port=9
  Bus Creator1 : BusCreator  Inputs=7
  Rate Limiter : RateLimiter  RisingSlewLimit=50  FallingSlewLimit=-50  SampleTimeMode=inherited
  Rate Limiter1 : RateLimiter  RisingSlewLimit=50  FallingSlewLimit=-50  SampleTimeMode=inherited
  Rate Limiter2 : RateLimiter  RisingSlewLimit=50  FallingSlewLimit=-50  SampleTimeMode=inherited
  Rate Limiter3 : RateLimiter  RisingSlewLimit=15  FallingSlewLimit=-15  SampleTimeMode=inherited
  Rate Limiter4 : RateLimiter  RisingSlewLimit=15  FallingSlewLimit=-15  SampleTimeMode=inherited
  Rate Limiter5 : RateLimiter  RisingSlewLimit=15  FallingSlewLimit=-15  SampleTimeMode=inherited
  Rate Limiter6 : RateLimiter  RisingSlewLimit=20  FallingSlewLimit=-20  SampleTimeMode=inherited
  Switch : Switch  Criteria=u2 ~= 0
  Out1 : Outport
  wires:
  In3/1 -> Switch/1
  Switch/1 -> Rate Limiter/1  "GuidanceForce_pct"
  In7/1 -> Rate Limiter4/1
  In8/1 -> Rate Limiter5/1
  In9/1 -> Rate Limiter6/1
  In4/1 -> Rate Limiter1/1
  In5/1 -> Rate Limiter2/1
  In6/1 -> Rate Limiter3/1
  GeneralGF/1 -> Switch/3
  Rate Limiter5/1 -> Bus Creator1/6  "DurationRight_pct"
  Rate Limiter/1 -> Bus Creator1/1  "GuidanceForce_pct"
  Rate Limiter4/1 -> Bus Creator1/5  "DurationLeft_pct"
  Rate Limiter3/1 -> Bus Creator1/4  "Timing_pct"
  Rate Limiter1/1 -> Bus Creator1/2  "AmplitudeLeft_pct"
  Rate Limiter6/1 -> Bus Creator1/7  "StepWidth_pct"
  Bus Creator1/1 -> Out1/1
  Rate Limiter2/1 -> Bus Creator1/3  "AmplitudeRight_pct"
  In2/1 -> Switch/2

== system LopesDevelopmentLibrary/GaitGenerationExtra/GaitParameters/StabilityInStance ==

== system LopesDevelopmentLibrary/GaitGenerationExtra/GaitParameters/StepHeight ==

== system LopesDevelopmentLibrary/GaitGenerationExtra/GaitParameters/StepLength ==

== system LopesDevelopmentLibrary/GaitGenerationExtra/GaitParameters/WeightShift ==

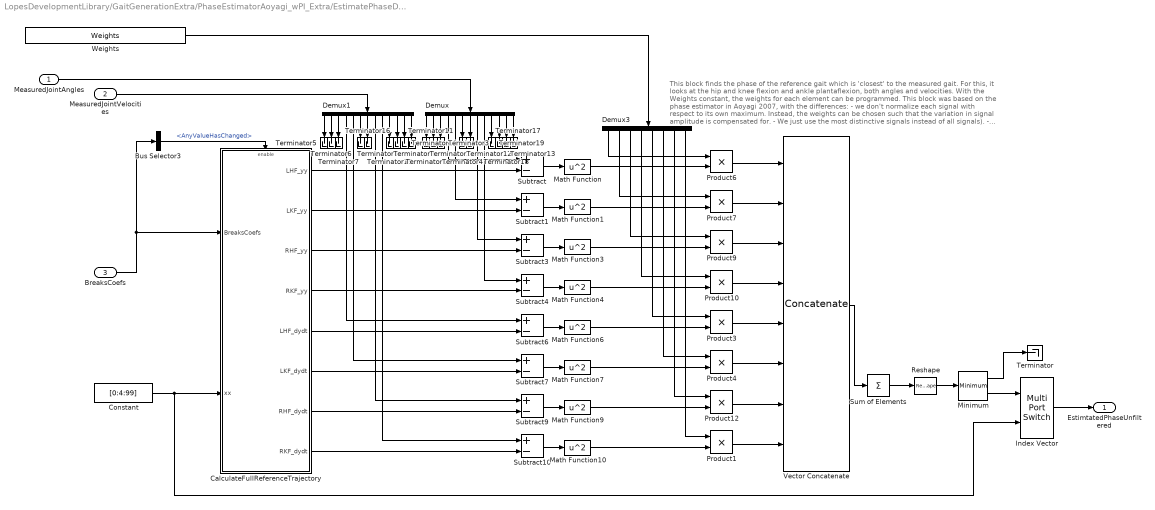
== system LopesDevelopmentLibrary/GaitGenerationExtra/PhaseEstimatorAoyagi_wPI_Extra/EstimatePhaseDirectlyAoyagi ==
  note: This block finds the phase of the reference gait which is 'closest' to the
      | measured gait. For this, it looks at the hip and knee flexion and ankle plantaflexion,
      | both angles and velocities. With the Weights constant, the weights for each element
      | can be programmed.
      | This block was based on the phase estimator in Aoyagi 2007, with the differences:
      | - we don't normalize each signal with respect to its own maximum. Instead, the weights
      | can be chosen such that the variation in signal amplitude is compensated for.
      | - We just use the most distinctive signals instead of all signals).
      | - The phase is expressed in percent  [0,100) instead of [0,1).
  MeasuredJointAngles : Inport
  MeasuredJointVelocities : Inport  Port=2
  BreaksCoefs : Inport  Port=3
  Bus Selector3 : BusSelector  OutputSignals=AnyValueHasChanged
  CalculateFullReferenceTrajectory : Subsystem
  Constant : Constant  Value=[0:4:99]
  Demux : Demux  Outputs=13
  Demux1 : Demux  Outputs=13
  Demux3 : Demux  Outputs=8
  Index Vector : MultiPortSwitch  Inputs=1
  Math Function{,1,3..4,6..7,9..10} (8 alike) : Math  Operator=square  SaturateOnIntegerOverflow=on
  Minimum : dspstat3/Minimum  fcn=Value and Index  reset=None  InputProcessing=Columns as channels (frame based)  indexBase=One  operateOver=Each column  Dimension=1  operation=minimum  roiEnable=off  roiType=Rectangles  roiPortion=Entire ROI  roiOutput=Individual statistics for each ROI  roiFlag=off  roundingMode=Floor  overflowMode=off
  Product{1,3..4,6..7,9..10,12} (8 alike) : Product  RndMeth=Zero
  Reshape : Reshape
  Subtract{,1,3..4,6..7,9..10} (8 alike) : Sum  Inputs=+-
  Sum of Elements : Sum  Inputs=+  CollapseMode=Specified dimension  CollapseDim=2
  Terminator{,1..13,15..19} (19 alike) : Terminator
  Vector Concatenate : Concatenate  NumInputs=8  Mode=Multidimensional array  ConcatenateDimension=2
  Weights : Constant  Value=Weights
  EstimtatedPhaseUnfiltered : Outport
  wires:
  Demux3/8 -> Product1/1
  Demux3/7 -> Product12/1
  Demux3/6 -> Product4/1
  Demux3/5 -> Product3/1
  Demux3/4 -> Product10/1
  Demux3/3 -> Product9/1
  Demux3/2 -> Product7/1
  Demux3/1 -> Product6/1
  Bus Selector3/1 -> CalculateFullReferenceTrajectory/Enable  "<AnyValueHasChanged>"
  CalculateFullReferenceTrajectory/8(RKF_dydt) -> Subtract10/2
  CalculateFullReferenceTrajectory/7(RHF_dydt) -> Subtract9/2
  CalculateFullReferenceTrajectory/6(LKF_dydt) -> Subtract7/2
  CalculateFullReferenceTrajectory/5(LHF_dydt) -> Subtract6/2
  CalculateFullReferenceTrajectory/4(RKF_yy) -> Subtract4/2
  CalculateFullReferenceTrajectory/3(RHF_yy) -> Subtract3/2
  CalculateFullReferenceTrajectory/2(LKF_yy) -> Subtract1/2
  CalculateFullReferenceTrajectory/1(LHF_yy) -> Subtract/2
  Reshape/1 -> Minimum/1
  Product1/1 -> Vector Concatenate/8
  Product12/1 -> Vector Concatenate/7
  Product3/1 -> Vector Concatenate/5
  Product4/1 -> Vector Concatenate/6
  Math Function10/1 -> Product1/2
  Math Function9/1 -> Product12/2
  Math Function7/1 -> Product4/2
  Math Function6/1 -> Product3/2
  Demux1/9 -> Subtract10/1
  Demux1/8 -> Subtract9/1
  Demux1/5 -> Subtract7/1
  Demux1/4 -> Subtract6/1
  Subtract10/1 -> Math Function10/1
  Subtract9/1 -> Math Function9/1
  Subtract7/1 -> Math Function7/1
  Subtract6/1 -> Math Function6/1
  MeasuredJointVelocities/1 -> Demux1/1
  Minimum/2 -> Index Vector/1
  Sum of Elements/1 -> Reshape/1
  Vector Concatenate/1 -> Sum of Elements/1
  Product10/1 -> Vector Concatenate/4
  Product9/1 -> Vector Concatenate/3
  Product6/1 -> Vector Concatenate/1
  Product7/1 -> Vector Concatenate/2
  Weights/1 -> Demux3/1
  Math Function4/1 -> Product10/2
  Math Function3/1 -> Product9/2
  Math Function1/1 -> Product7/2
  Math Function/1 -> Product6/2
  Subtract4/1 -> Math Function4/1
  Subtract3/1 -> Math Function3/1
  Subtract1/1 -> Math Function1/1
  Subtract/1 -> Math Function/1
  Demux/9 -> Subtract4/1
  Demux/8 -> Subtract3/1
  Index Vector/1 -> EstimtatedPhaseUnfiltered/1
  BreaksCoefs/1 -> CalculateFullReferenceTrajectory/1(BreaksCoefs), Bus Selector3/1
  MeasuredJointAngles/1 -> Demux/1
  Constant/1 -> CalculateFullReferenceTrajectory/2(xx), Index Vector/2
  Demux/4 -> Subtract/1
  Demux/5 -> Subtract1/1
  Minimum/1 -> Terminator/1
  Demux1/6 -> Terminator8/1
  Demux1/3 -> Terminator7/1
  Demux1/2 -> Terminator6/1
  Demux1/1 -> Terminator5/1
  Demux/1 -> Terminator1/1
  Demux/2 -> Terminator2/1
  Demux/3 -> Terminator3/1
  Demux/6 -> Terminator4/1
  Demux1/10 -> Terminator15/1
  Demux1/11 -> Terminator9/1
  Demux/10 -> Terminator19/1
  Demux1/12 -> Terminator10/1
  Demux1/13 -> Terminator11/1
  Demux1/7 -> Terminator16/1
  Demux/13 -> Terminator13/1
  Demux/12 -> Terminator18/1
  Demux/11 -> Terminator17/1
  Demux/7 -> Terminator12/1

== system LopesDevelopmentLibrary/GaitGenerationExtra/PhaseEstimatorAoyagi_wPI_Extra/PhaseFilterAoyagi ==
  note: "'PI-controller". Makes sure that the phase error will eventually
      | go to zero. Hopefully this will make the system better. However, the integral is
      | limited to -20..20 to prevent problems when a non-walking state is detected.
  note: This filter is based on the filter described in Aoyagi 2007.
      | It differs on the following points:
      | - Range [0,100) %, not [0,1) scale.
      | - Different implementation of wrap around integration (Aoyagi uses a resettable integrator; I use a mod 100)
      | - AoyagiFilterGain should be the same as in the paper (the error is 100 times larger than Aoyagi's, but so is
      |    the range of the integration). I found however that 2.5 for a gain [Aoyagi 2007] is quite low.
      | - In the figure in the paper no saturation is shown, but in the text they tell that there is saturation. I use it
      |    here too (so that phase cannot go backwards and cannot go rise too fast).
  EstimatedPhaseUnfiltered : Inport
  ReferenceStrideTime : Inport  Port=2
  ResetHighActive : Inport  Port=3
  x0 : Inport  Port=4
  FinalState : Inport  Port=5
  AoyagiFilterGain : Gain  Gain=AoyagiFilterGain
  CalculateStridesPerSec : Math  Operator=reciprocal  SaturateOnIntegerOverflow=on
  Constant : Constant  Value=inf
  Constant1 : Constant  Value=20
  Divide : Product  Inputs=/*
  Gain : Gain  Gain=3
  Gain1 : Gain  Gain=0.2
  IntegralTimeConstant : Constant  Value=AoyagiIntegralTimeConstant
  Integrator : Integrator  ExternalReset=level  InitialConditionSource=external
  Integrator1 : Integrator  ExternalReset=level  LimitOutput=on  UpperSaturationLimit=20  LowerSaturationLimit=-20
  PhaseWrapper : LopesDevelopmentLibrary/Various/PhaseWrapper
  Product : Product
  Saturation Dynamic : simulink/Discontinuities/Saturation Dynamic  OutMin=[]  OutMax=[]  OutDataTypeStr=Inherit: Same as second input  OutDataType=fixdt(1, 16)  OutScaling=2^-10  DoSatur=off
  Saturation Dynamic1 : simulink/Discontinuities/Saturation Dynamic  OutMin=[]  OutMax=[]  OutDataTypeStr=Inherit: Same as second input  OutDataType=fixdt(1, 16)  OutScaling=2^-10  DoSatur=off
  Sum : Sum  Inputs=|+-
  Sum1 : Sum  Inputs=++|
  Sum2 : Sum  Inputs=++|
  ToPercentPerSec : Gain  Gain=100
  Wrap_Min50_Plus50 : Subsystem
  EstimatedPhase : Outport
  EstimatedPhaseRate : Outport  Port=2
  wires:
  Product/1 -> Saturation Dynamic1/3
  Saturation Dynamic1/1 -> Integrator/1
  FinalState/1 -> Product/2
  Constant1/1 -> Product/1
  Constant/1 -> Saturation Dynamic1/1
  Saturation Dynamic/1 -> Saturation Dynamic1/2
  x0/1 -> Integrator/3
  Sum2/1 -> Sum1/1
  Integrator1/1 -> Sum2/1
  Divide/1 -> Integrator1/1
  IntegralTimeConstant/1 -> Divide/1
  Gain/1 -> Saturation Dynamic/1
  Gain1/1 -> Saturation Dynamic/3
  ReferenceStrideTime/1 -> CalculateStridesPerSec/1
  Sum/1 -> Wrap_Min50_Plus50/1(In)
  Wrap_Min50_Plus50/1(Out) -> AoyagiFilterGain/1
  CalculateStridesPerSec/1 -> ToPercentPerSec/1
  PhaseWrapper/1 -> EstimatedPhase/1, Sum/2
  ToPercentPerSec/1 -> Gain/1, Gain1/1, Sum2/2
  AoyagiFilterGain/1 -> Divide/2, Sum1/2
  Sum1/1 -> Saturation Dynamic/2
  EstimatedPhaseUnfiltered/1 -> Sum/1
  Integrator/1 -> PhaseWrapper/1
  ResetHighActive/1 -> Integrator/2, Integrator1/2

== system LopesDevelopmentLibrary/GaitPhaseDetection/Gait Phase Detection with Wrapper/Data selection ==
  Cart_pos : Inport
  Treadmill : Inport  Port=2
  Angle_l : Subsystem
  Angle_r : Subsystem
  Selector : Selector  InputPortWidth=21  IndexOptions=Index vector (dialog)  Indices=[11]  OutputSizes=1
  Selector1 : Selector  InputPortWidth=21  IndexOptions=Index vector (dialog)  Indices=[20]  OutputSizes=1
  Selector10 : Selector  InputPortWidth=21  IndexOptions=Index vector (dialog)  Indices=[16 17 18]  OutputSizes=1
  Selector11 : Selector  InputPortWidth=21  IndexOptions=Index vector (dialog)  Indices=[13 14 15]  OutputSizes=1
  Selector2 : Selector  InputPortWidth=21  IndexOptions=Index vector (dialog)  Indices=[19]  OutputSizes=1
  Selector3 : Selector  InputPortWidth=21  IndexOptions=Index vector (dialog)  Indices=[10]  OutputSizes=1
  Selector4 : Selector  InputPortWidth=7  IndexOptions=Index vector (dialog)  Indices=[2]  OutputSizes=1
  Selector5 : Selector  InputPortWidth=21  IndexOptions=Index vector (dialog)  Indices=[10 11 12]  OutputSizes=1
  Selector6 : Selector  InputPortWidth=21  IndexOptions=Index vector (dialog)  Indices=[7 8 9]  OutputSizes=1
  Selector7 : Selector  InputPortWidth=21  IndexOptions=Index vector (dialog)  Indices=[4 5 6]  OutputSizes=1
  Selector9 : Selector  InputPortWidth=21  IndexOptions=Index vector (dialog)  Indices=[19 20 21]  OutputSizes=1
  ankle_y_l : Outport
  ankle_x_l : Outport  Port=2
  angle_knee_l : Outport  Port=3
  ankle_y_r : Outport  Port=4
  ankle_x_r : Outport  Port=5
  angle_knee_r : Outport  Port=6
  Treadmill speed : Outport  Port=7
  wires:
  Angle_r/1(angle_r) -> angle_knee_r/1
  Angle_l/1(angle_l) -> angle_knee_l/1
  Selector11/1 -> Angle_r/3(hip)
  Selector9/1 -> Angle_r/1(ankle)
  Selector10/1 -> Angle_r/2(knee)
  Selector7/1 -> Angle_l/3(hip)
  Selector6/1 -> Angle_l/2(knee)
  Selector5/1 -> Angle_l/1(ankle)
  Cart_pos/1 -> Selector/1, Selector3/1, Selector1/1, Selector2/1, Selector6/1, Selector7/1, Selector9/1, Selector11/1, Selector10/1, Selector5/1
  Selector/1 -> ankle_y_l/1
  Selector1/1 -> ankle_y_r/1
  Selector4/1 -> Treadmill speed/1
  Selector3/1 -> ankle_x_l/1
  Treadmill/1 -> Selector4/1
  Selector2/1 -> ankle_x_r/1

== system LopesDevelopmentLibrary/GaitPhaseDetection/Gait Phase Detection with Wrapper/LeftLegWalking ==
  note: Right foot detection
      | 1 = stance phase
      | 2 = swing phase
  ankle_y_r_dot : Inport
  ankle_x_r_dot : Inport  Port=2
  knee_angle_dot : Inport  Port=3
  belt_speed : Inport  Port=4
  Add2 : Sum  OutDataTypeStr=double
  Heel strike detection : Subsystem
  Heel strike_safety : Subsystem
  Logical Operator2 : Logic  Operator=OR  AllPortsSameDT=off  OutDataTypeStr=boolean
  Sample and Hold2 : dspsigops/Sample and Hold  trig=Rising edge  initCond=1  latchinput=off
  Toe-off detection : Subsystem
  Left : Outport  OutDataTypeStr=double
  wires:
  Sample and Hold2/1 -> Left/1
  Logical Operator2/1 -> Add2/1
  Add2/1 -> Sample and Hold2/Trigger, Sample and Hold2/1
  ankle_x_r_dot/1 -> Heel strike_safety/1(ankle_x_dot), Heel strike detection/2(ankle_x_dot), Toe-off detection/1(ankle_x_dot)  "ankle_x_dot"
  ankle_y_r_dot/1 -> Heel strike detection/1(ankle_y_dot)  "ankle_y_dot"
  Heel strike detection/1(Heel_strike) -> Logical Operator2/1
  Toe-off detection/1(Toe_off) -> Add2/2
  belt_speed/1 -> Heel strike_safety/2(belt_speed)
  Heel strike_safety/1(Heel_strike_safety) -> Logical Operator2/2
  knee_angle_dot/1 -> Toe-off detection/2(knee_angle_dot)
